simulink model "Drone_smc_2018"  (R2018a)
settings: Solver=FixedStepAuto  StartTime=0.0  StopTime=T  FixedStep=Ts  RelTol=1e-3
values from neighbouring files (symbols this model uses):
  kd_d = 8    [drone_parameters.m]
  ki_d = 0.1    [drone_parameters.m]
  kp_d = 7    [drone_parameters.m]
  si_d = 1*pi/180    (= 0.0174532925199)    [drone_parameters.m]
  T = 50    [drone_parameters.m]
  x_d = 20    [drone_parameters.m]
  y_d = 65    [drone_parameters.m]
  z_d = 50    [drone_parameters.m]
undefined symbols (not defined in the file or in its folder): attitude_ctrl, droneOrientation, droneparam, dronePos, height_input
settings Model: Creator=saad  LastModifiedBy=Anay Panshikar

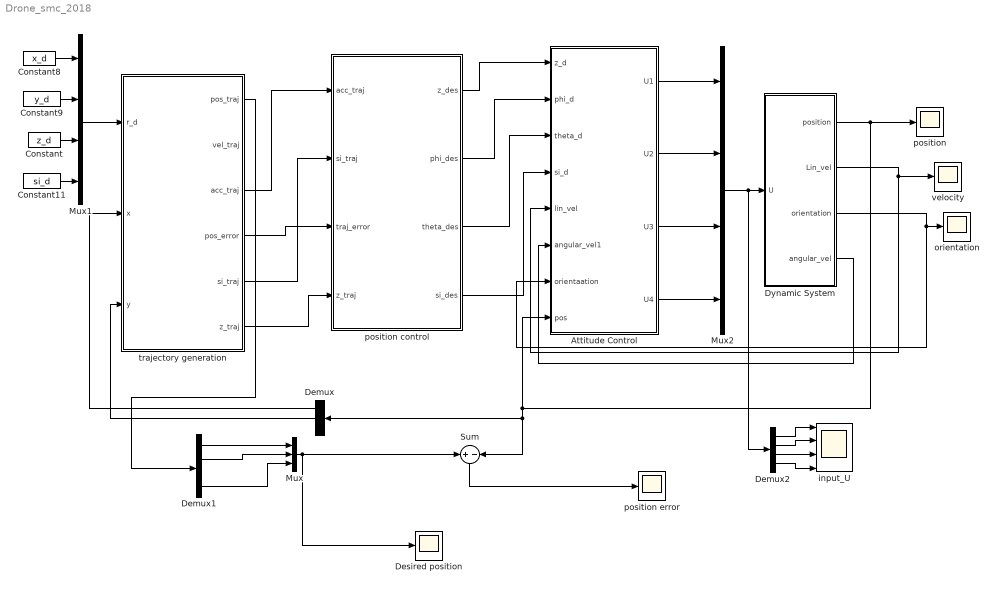
== system Drone_smc_2018 ==
  Attitude Control : Subsystem
  Constant : Constant  Value=z_d
  Constant11 : Constant  Value=si_d
  Constant8 : Constant  Value=x_d
  Constant9 : Constant  Value=y_d
  Demux : Demux  Outputs=3
  Demux1 : Demux
  Demux2 : Demux
  "Desired position " : Scope
  "Dynamic System " : Subsystem
  Mux : Mux  Inputs=3
  Mux1 : Mux
  Mux2 : Mux
  Sum : Sum  Inputs=+-
  input_U : Scope  NumInputPorts=4
  orientation : Scope
  "position " : Scope
  position control : Subsystem
  position error : Scope
  trajectory generation : Subsystem
  "velocity " : Scope
  wires:
  position control/4(si_des) -> Attitude Control/4(si_d)
  position control/3(theta_des) -> Attitude Control/3(theta_d)
  Mux2/1 -> Demux2/1, "Dynamic System "/1(U)
  "Dynamic System "/2(Lin_vel) -> Attitude Control/5(lin_vel), "velocity "/1
  position control/2(phi_des) -> Attitude Control/2(phi_d)
  "Dynamic System "/1("position ") -> Sum/2, Demux/1, Attitude Control/8(pos), "position "/1
  "Dynamic System "/3(orientation) -> Attitude Control/7(orientaation), orientation/1
  Constant9/1 -> Mux1/2
  Mux1/1 -> trajectory generation/1(r_d)
  Constant8/1 -> Mux1/1
  Constant/1 -> Mux1/3
  Constant11/1 -> Mux1/4
  trajectory generation/4(pos_error) -> position control/3(traj_error)
  trajectory generation/5(si_traj) -> position control/2(si_traj)
  Demux/1 -> trajectory generation/2(x)
  Demux/2 -> trajectory generation/3(y)
  trajectory generation/6(z_traj) -> position control/4(z_traj)
  position control/1(z_des) -> Attitude Control/1(z_d)
  "Dynamic System "/4(angular_vel) -> Attitude Control/6(angular_vel1)
  Attitude Control/1(U1) -> Mux2/1
  Attitude Control/2(U2) -> Mux2/2
  Attitude Control/3(U3) -> Mux2/3
  Attitude Control/4(U4) -> Mux2/4
  Sum/1 -> position error/1
  trajectory generation/1(pos_traj) -> Demux1/1
  Demux1/1 -> Mux/1
  Demux1/2 -> Mux/2
  Demux1/4 -> Mux/3
  Mux/1 -> "Desired position "/1, Sum/1
  Demux2/4 -> input_U/4
  Demux2/3 -> input_U/3
  Demux2/2 -> input_U/2
  Demux2/1 -> input_U/1
  trajectory generation/3(acc_traj) -> position control/1(acc_traj)

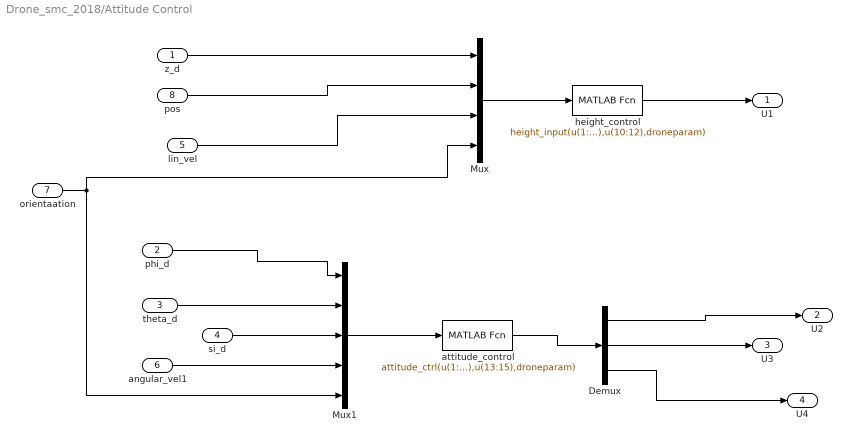
== system Drone_smc_2018/Attitude Control ==
  z_d : Inport
  phi_d : Inport  Port=2
  theta_d : Inport  Port=3
  si_d : Inport  Port=4
  lin_vel : Inport  Port=5
  angular_vel1 : Inport  Port=6
  orientaation : Inport  Port=7
  pos : Inport  Port=8
  Demux : Demux  Outputs=3
  Mux : Mux
  Mux1 : Mux  Inputs=5
  attitude_control : MATLABFcn  MATLABFcn=attitude_ctrl(u(1:3),u(4:6),u(7:9),u(10:12),u(13:15),droneparam)  OutputDimensions=3
  height_control : MATLABFcn  MATLABFcn=height_input(u(1:3),u(4:6),u(7:9),u(10:12),droneparam)  OutputDimensions=1
  U1 : Outport  VectorParamsAs1DForOutWhenUnconnected=off
  U2 : Outport  Port=2  VectorParamsAs1DForOutWhenUnconnected=off
  U3 : Outport  Port=3  VectorParamsAs1DForOutWhenUnconnected=off
  U4 : Outport  Port=4  VectorParamsAs1DForOutWhenUnconnected=off
  wires:
  z_d/1 -> Mux/1
  lin_vel/1 -> Mux/3
  orientaation/1 -> Mux1/5, Mux/4
  pos/1 -> Mux/2
  theta_d/1 -> Mux1/2
  si_d/1 -> Mux1/3
  angular_vel1/1 -> Mux1/4
  Mux/1 -> height_control/1
  phi_d/1 -> Mux1/1
  Mux1/1 -> attitude_control/1
  attitude_control/1 -> Demux/1
  Demux/1 -> U2/1
  Demux/3 -> U4/1
  Demux/2 -> U3/1
  height_control/1 -> U1/1

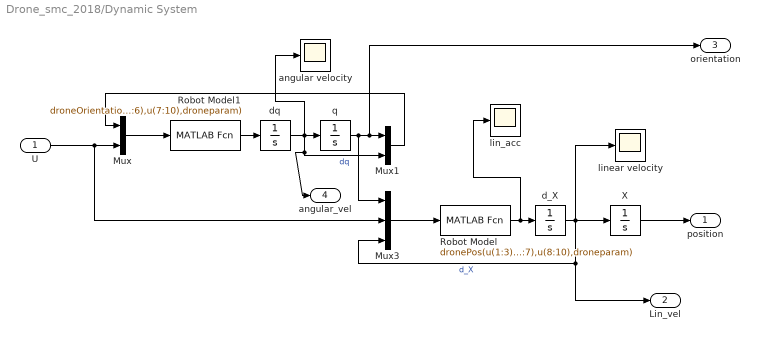
== system Drone_smc_2018/Dynamic System  ==
  U : Inport
  Mux : Mux  Inputs=2
  Mux1 : Mux  Inputs=2
  Mux3 : Mux  Inputs=3
  Robot Model : MATLABFcn  MATLABFcn=dronePos(u(1:3),u(4:7),u(8:10),droneparam)  OutputDimensions=3
  Robot Model1 : MATLABFcn  MATLABFcn=droneOrientation(u(1:3),u(4:6),u(7:10),droneparam)  OutputDimensions=3
  X : Integrator  InitialCondition=droneparam.X0
  angular velocity : Scope
  d_X : Integrator  InitialCondition=droneparam.X0
  dq : Integrator  InitialCondition=droneparam.q0
  lin_acc : Scope
  "linear velocity " : Scope
  q : Integrator  InitialCondition=droneparam.q0
  "position " : Outport  VectorParamsAs1DForOutWhenUnconnected=off
  Lin_vel : Outport  Port=2  VectorParamsAs1DForOutWhenUnconnected=off
  orientation : Outport  Port=3  VectorParamsAs1DForOutWhenUnconnected=off
  angular_vel : Outport  Port=4  VectorParamsAs1DForOutWhenUnconnected=off
  wires:
  Mux3/1 -> Robot Model/1
  q/1 -> Mux3/1, orientation/1, Mux1/1
  X/1 -> "position "/1
  U/1 -> Mux3/2, Mux/2
  Mux/1 -> Robot Model1/1
  Mux1/1 -> Mux/1
  dq/1 -> angular velocity/1, angular_vel/1, Mux1/2, q/1  "dq"
  Robot Model1/1 -> dq/1
  Robot Model/1 -> lin_acc/1, d_X/1
  d_X/1 -> Lin_vel/1, Mux3/3, "linear velocity "/1, X/1  "d_X"

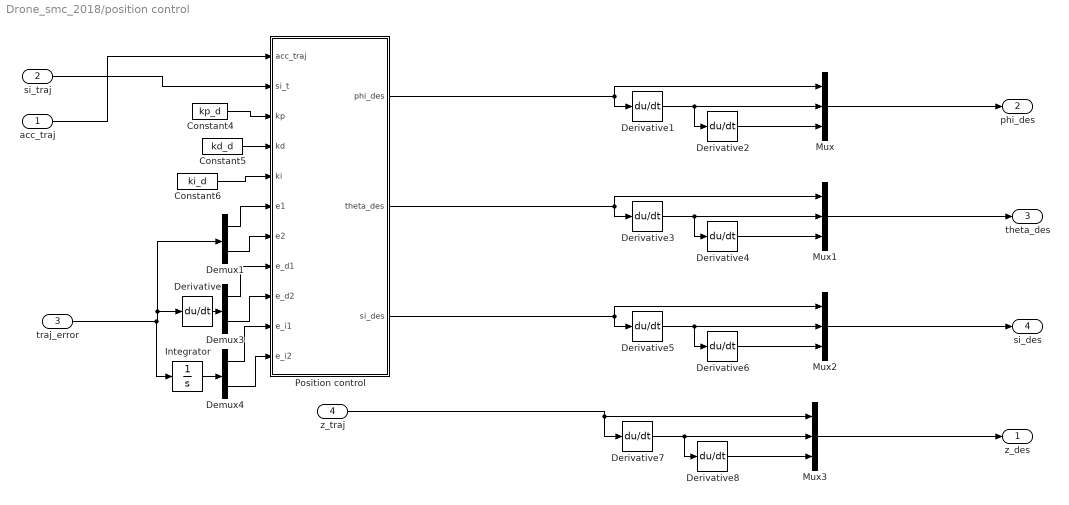
== system Drone_smc_2018/position control ==
  acc_traj : Inport
  si_traj : Inport  Port=2
  traj_error : Inport  Port=3
  z_traj : Inport  Port=4
  Constant4 : Constant  Value=kp_d
  Constant5 : Constant  Value=kd_d
  Constant6 : Constant  Value=ki_d
  Demux1 : Demux  Outputs=2
  Demux3 : Demux  Outputs=2
  Demux4 : Demux  Outputs=2
  Derivative{,1..8} (9 alike) : Derivative
  Integrator : Integrator
  Mux{,1..3} (4 alike) : Mux  Inputs=3
  Position control : MATLAB Function  TreatAsAtomicUnit=on
  z_des : Outport  VectorParamsAs1DForOutWhenUnconnected=off
  phi_des : Outport  Port=2  VectorParamsAs1DForOutWhenUnconnected=off
  theta_des : Outport  Port=3  VectorParamsAs1DForOutWhenUnconnected=off
  si_des : Outport  Port=4  VectorParamsAs1DForOutWhenUnconnected=off
  wires:
  si_traj/1 -> Position control/2(si_t)
  Demux3/2 -> Position control/9(e_d2)
  traj_error/1 -> Integrator/1, Demux1/1, Derivative/1
  Demux4/2 -> Position control/11(e_i2)
  Demux1/2 -> Position control/7(e2)
  Demux1/1 -> Position control/6(e1)
  Constant6/1 -> Position control/5(ki)
  Constant4/1 -> Position control/3(kp)
  Constant5/1 -> Position control/4(kd)
  Position control/1(phi_des) -> Mux/1, Derivative1/1
  Integrator/1 -> Demux4/1
  Demux4/1 -> Position control/10(e_i1)
  Derivative/1 -> Demux3/1
  Demux3/1 -> Position control/8(e_d1)
  Derivative1/1 -> Derivative2/1, Mux/2
  Derivative2/1 -> Mux/3
  Mux/1 -> phi_des/1
  Derivative4/1 -> Mux1/3
  Mux1/1 -> theta_des/1
  Position control/2(theta_des) -> Mux1/1, Derivative3/1
  Derivative3/1 -> Derivative4/1, Mux1/2
  Derivative6/1 -> Mux2/3
  Mux2/1 -> si_des/1
  Position control/3(si_des) -> Mux2/1, Derivative5/1
  Derivative5/1 -> Derivative6/1, Mux2/2
  z_traj/1 -> Mux3/1, Derivative7/1
  Derivative7/1 -> Derivative8/1, Mux3/2
  Derivative8/1 -> Mux3/3
  Mux3/1 -> z_des/1
  acc_traj/1 -> Position control/1(acc_traj)

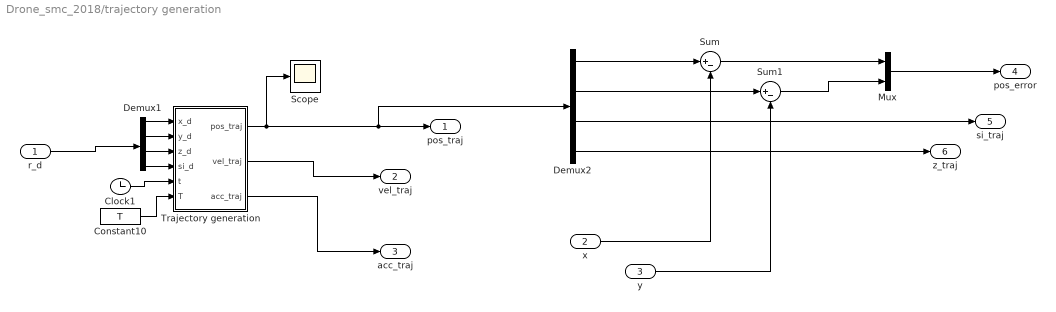
== system Drone_smc_2018/trajectory generation ==
  r_d : Inport
  x : Inport  Port=2
  y : Inport  Port=3
  Clock1 : Clock
  Constant10 : Constant  Value=T
  Demux1 : Demux
  Demux2 : Demux
  Mux : Mux  Inputs=2
  Scope : Scope
  Sum : Sum  Inputs=|+-
  Sum1 : Sum  Inputs=|+-
  Trajectory generation : MATLAB Function  TreatAsAtomicUnit=on
  pos_traj : Outport  VectorParamsAs1DForOutWhenUnconnected=off
  vel_traj : Outport  Port=2  VectorParamsAs1DForOutWhenUnconnected=off
  acc_traj : Outport  Port=3  VectorParamsAs1DForOutWhenUnconnected=off
  pos_error : Outport  Port=4  VectorParamsAs1DForOutWhenUnconnected=off
  si_traj : Outport  Port=5  VectorParamsAs1DForOutWhenUnconnected=off
  z_traj : Outport  Port=6  VectorParamsAs1DForOutWhenUnconnected=off
  wires:
  Clock1/1 -> Trajectory generation/5(t)
  Demux1/2 -> Trajectory generation/2(y_d)
  Demux1/1 -> Trajectory generation/1(x_d)
  Demux1/4 -> Trajectory generation/4(si_d)
  r_d/1 -> Demux1/1
  Constant10/1 -> Trajectory generation/6(T)
  Demux1/3 -> Trajectory generation/3(z_d)
  Trajectory generation/2(vel_traj) -> vel_traj/1
  Trajectory generation/3(acc_traj) -> acc_traj/1
  Trajectory generation/1(pos_traj) -> Scope/1, Demux2/1, pos_traj/1
  x/1 -> Sum/2
  Demux2/1 -> Sum/1
  Demux2/2 -> Sum1/1
  y/1 -> Sum1/2
  Sum/1 -> Mux/1
  Sum1/1 -> Mux/2
  Mux/1 -> pos_error/1
  Demux2/3 -> si_traj/1
  Demux2/4 -> z_traj/1

== matlab function Drone_smc_2018/trajectory generation/Trajectory generation ==
  data: x_d input; pos_traj output; y_d input; z_d input; si_d input; t input; T input; vel_traj output; acc_traj output
function [pos_traj,vel_traj,acc_traj] = fcn(x_d,y_d,z_d,si_d,t,T)
    x_traj = x_d*t^2/T^2;
    y_traj = y_d*t^2/T^2;
    si_traj = si_d*t^2/T^2;
    z_traj = z_d*t^2/T^2;
    
    dx_traj = 2*x_d*t/T^2;
    dy_traj = 2*y_d*t/T^2;
    dsi_traj = 2*si_d*t/T^2;
    dz_traj = 2*z_d*t/T^2;
    
    ddx_traj = 2*x_d/T^2;
    ddy_traj = 2*y_d/T^2;
    ddsi_traj = 2*si_d/T^2;
    ddz_traj = 2*z_d/T^2;
    
    pos_traj = [x_traj y_traj si_traj z_traj];
    
    vel_traj = [dx_traj dy_traj dsi_traj dz_traj];
    
    acc_traj = [ddx_traj ddy_traj ddsi_traj ddz_traj];
end

== matlab function Drone_smc_2018/position control/Position control ==
  data: acc_traj input; si_t input; kp input; kd input; ki input; phi_des output; e1 input; theta_des output; e2 input; e_d1 input; si_des output; e_d2 input; e_i1 input; e_i2 input
function [phi_des,theta_des,si_des] = fcn(acc_traj, si_t,kp,kd,ki,e1,e2,e_d1,e_d2,e_i1,e_i2)
        e = [e1 e2];
        e_d = [e_d1 e_d2];
        e_i = [e_i1 e_i2];
   
    s1 = e_d1 + kp*e1;
    s2 = e_d2 + kp*e2;
    axstar = acc_traj(1);
    aystar = acc_traj(2);
    
    ddr_des = [axstar aystar] + kd*e_d + [sat(s1) sat(s2)] + 10.*[s1 s2];
    
    phi_des = (ddr_des(1)*sin(si_t) - ddr_des(2)*cos(si_t))/9.8;
    
    theta_des = (ddr_des(1)*cos(si_t) + ddr_des(2)*sin(si_t))/9.8;
    
    si_des = si_t;
end

function Y=sat(s)
% % sat is the saturation function with unit limits and unit slope.
%     if s>1
%         Y=1;
%     elseif s<-1 
%         Y=-1;
%     else 
%         Y=s;
%     end
    Y = s./(abs(s)+0.001);
end
